simulink model "sm_cable_robot"  (R2021b)
settings: Solver=ode45  StartTime=0.0  StopTime=10  MaxStep=0.01  RelTol=1e-3  EnableMultiTasking=on
model workspace: external: MATLAB File sm_cable_robot_parameters.m (data not in the file)
values from neighbouring files (symbols this model uses):
  g = 9.80665    [sm_cable_robot_parameters.m]
undefined symbols (not defined in the file or in its folder): ball, frame, Hand, Left, mover, Right, X, Y, Z
libraries: sm_lib x12, nesl_utility x7, sm_cable_robot_lib x4
Description:
  | Cable Robot
settings Model: Creator=The MathWorks, Inc.  LastModifiedBy=The MathWorks, Inc.
settings SolverCC: AlgebraicLoopSolver=TrustRegion  MinimalZcImpactIntegration=on
settings DataIOCC: LimitDataPoints=on  ReturnWorkspaceOutputs=off
settings OptimizationCC: LifeSpan=inf
settings DebuggingCC: AllowSymbolicDim=off  SFUnexpectedBacktrackingDiag=warning  SFNoUnconditionalDefaultTransitionDiag=warning  SFExecutionAtInitializationDiag=none  SFMachineParentedDataDiag=warning  ArithmeticOperatorsInVariantConditions=warning
settings SFSimCC: SimUseLocalCustomCode=off
settings RTWCC: RTWUseLocalCustomCode=off
settings CodeAppCC: StateflowObjectComments=on
settings GRTTargetCC: TargetLangStandard=C89/C90 (ANSI)
settings ConfigComp: CovMetricSettings=dw  CovSaveCumulativeToWorkspaceVar=on  CovSaveSingleToWorkspaceVar=on  CovExternalEMLEnable=off  CovSFcnEnable=off
settings SimscapeCC: SimscapeNominalValues="[{\"value\":\"10\",\"unit\":\"V\"},{\"value\":\"1\",\"unit\":\"A\"},{\"value\":\"10\",\"unit\":\"N*m\"},{\"value\":\"10\",\"unit\":\"bar\"},{\"value\":\"100\",\"unit\":\"kJ/kg\"},{\"value\":\"1\",\"unit\":\"kW\"},{\"value\":\"300\",\"unit\":\"K\"},{\"value\":\"100\",\"unit\":\"cm^3/s\"},{\"value\":\"1\",\"unit\":\"kN\"},{\"value\":\"1\",\"unit\":\"g/cm^3\"},{\"value\":\"1\",\"unit\":\"l\"},{\"value\":\"1\",\"unit\":\"cm^2\"},{\"value\":\"60\",\"unit\":\"Hz\"}]"  SimscapeLogType=all  SimscapeLogName=simlog_sm_cable_robot  SimscapeLogDataHistory=10000
settings ConfigurationSet: Description=SimMechanics 2G
settings DiagnosticsConfigSet: SimMechanicsRigidlyBoundBlock=none
settings ExplorerConfigSet: InternalSimMechanicsExplorerSettings="<ExplorerConfiguration><canonicalview>default</canonicalview><AnimationSetting><BasePlaybackSpeed>1.0</BasePlaybackSpeed><PlaybackSpeedFactor>0.5</PlaybackSpeedFactor></AnimationSetting><TilePanel><TileInfo><Tiles Columns=\"2\" Count=\"4\" Rows=\"2\"><Column Weight=\"0.4996\"/><Column Weight=\"0.5004\"/><Row Weight=\"0.5\"/><Row Weight=\"0.5\"/><Tile Height=\"1\" Width=\"1\" X=\"0\" Y=\"0\"/><Tile Height=\"1\" Width=\"1\" X=\"0\" Y=\"1\"/><Tile Height=\"1\" Width=\"1\" X=\"1\" Y=\"0\"/><Tile Height=\"1\" Width=\"1\" X=\"1\" Y=\"1\"/></Tiles></TileInfo><SceneInfo><SceneViewer><BGColor><R>0.60000002384185791</R><G>0.60000002384185791</G><B>0.60000002384185791</B></BGColor><Camera><DoPerspective>on</DoPerspective><Position><X>0</X><Y>0</Y><Z>1.80000000000000004</Z></Position><Center><X>0</X><Y>0</Y><Z>0.6835266900559267</Z></Center><Up><X>0</X><Y>1</Y><Z>0</Z></Up><ViewLimDist>1</ViewLimDist><YLim>0.466307658154998583</YLim><XLim>0.599116801300409563</XLim></Camera></SceneViewer><SceneViewer><BGColor><R>0.60000002384185791</R><G>0.60000002384185791</G><B>0.60000002384185791</B></BGColor><Camera><DoPerspective>on</DoPerspective><Position><X>-0.869999999999999996</X><Y>-0.719999999999999973</Y><Z>1</Z></Position><Center><X>0.720937841330330564</X><Y>0.696383532720419751</Y><Z>0.00254680794336636929</Z></Center><Up><X>0.316740818644561883</X><Y>0.281988691207070763</Y><Z>0.905625547252116636</Z></Up><ViewLimDist>1</ViewLimDist><YLim>0.466307658154998583</YLim><XLim>0.599116801300409563</XLim></Camera></SceneViewer><SceneViewer><BGColor><R>0.60000002384185791</R><G>0.60000002384185791</G><B>0.60000002384185791</B></BGColor><Camera><DoPerspective>on</DoPerspective><Position><X>2.03939800918097314</X><Y>9.95798776770584482e-09</Y><Z>0.494999989241745375</Z></Position><Center><X>0.644699031710575188</X><Y>9.95798776770584482e-09</Y><Z>0.494999989241745375</Z></Center><Up><X>-0</X><Y>0</Y><Z>1</Z></Up><ViewLimDist>1</ViewLimDist><YLim>0.466307658154998583</YLim><XLim>0.599116801300409563</XLim></Camera></SceneViewer><SceneViewer><BGColor><R>0.60000002384185791</R><G>0.60000002384185791</G><B>0.60000002384185791</B></BGColor><Camera><DoPerspective>on</DoPerspective><Position><X>1.69344100606403369</X><Y>-0.966528451082007023</Y><Z>0.938335299313491245</Z></Position><Center><X>0.749070842638739132</X><Y>-0.395339740352455893</Y><Z>0.516094349779432804</Z></Center><Up><X>-0.304859850331606563</X><Y>0.186390498904929286</Y><Z>0.933980221189807835</Z></Up><ViewLimDist>1</ViewLimDist><YLim>0.466307658154998583</YLim><XLim>0.599116801300409563</XLim></Camera></SceneViewer></SceneInfo></TilePanel><MechEditorPanel><Cameras><Camera><Id>Camera1</Id><Value><Name>Overhead</Name><NativeCamera><PositionKeyframeSet><Keyframe><Time>+0.0000000000000000e+00</Time><Value><X>+0.0000000000000000e+00</X><Y>+0.0000000000000000e+00</Y><Z>+1.8000000000000000e+00</Z></Value></Keyframe></PositionKeyframeSet><CenterKeyframeSet><Keyframe><Time>+0.0000000000000000e+00</Time><Value><X>+0.0000000000000000e+00</X><Y>+0.0000000000000000e+00</Y><Z>+6.8352669005592670e-01</Z></Value></Keyframe></CenterKeyframeSet><UpVectorKeyframeSet><Keyframe><Time>+0.0000000000000000e+00</Time><Value><X>+0.0000000000000000e+00</X><Y>+1.0000000000000000e+00</Y><Z>+0.0000000000000000e+00</Z></Value></Keyframe></UpVectorKeyframeSet></NativeCamera></Value></Camera><Camera><Id>Camera2</Id><Value><Name>Swivel Pulley</Name><NativeCamera><PositionKeyframeSet><Keyframe><Time>+0.0000000000000000e+00</Time><Value><X>-8.7000000000000000e-01</X><Y>-7.1999999999999997e-01</Y><Z>+1.0000000000000000e+00</Z></Value></Keyframe></PositionKeyframeSet><CenterKeyframeSet><Keyframe><Time>+0.0000000000000000e+00</Time><Value><X>+7.2093784133033056e-01</X><Y>+6.9638353272041975e-01</Y><Z>+2.5468079433663693e-03</Z></Value></Keyframe></CenterKeyframeSet><UpVectorKeyframeSet><Keyframe><Time>+0.0000000000000000e+00</Time><Value><X>+3.1674081864456188e-01</X><Y>+2.8198869120707076e-01</Y><Z>+9.0562554725211664e-01</Z></Value></Keyframe></UpVectorKeyframeSet></NativeCamera></Value></Camera><Camera><Id>Camera3</Id><Value><Name>Flyover</Name><NativeCamera><PositionKeyframeSet><Keyframe><Time>+0.0000000000000000e+00</Time><Value><X>+1.6934410060640337e+00</X><Y>-9.6652845108200702e-01</Y><Z>+9.3833529931349124e-01</Z></Value></Keyframe><Keyframe><Time>+4.9990750394185373e+00</Time><Value><X>+8.7196584858736648e-01</X><Y>+7.5039304919046734e-01</Y><Z>+1.0201392219856453e+00</Z></Value></Keyframe><Keyframe><Time>+6.7557213998445649e+00</Time><Value><X>+1.0978317870949922e-01</X><Y>+1.0441353295504237e+00</Y><Z>+6.6281255365999214e-01</Z></Value></Keyframe><Keyframe><Time>+1.0000000000000000e+01</Time><Value><X>-1.7603692267125191e+00</X><Y>+1.0439399563553646e+00</Y><Z>+9.9074072437996419e-01</Z></Value></Keyframe></PositionKeyframeSet><CenterKeyframeSet><Keyframe><Time>+0.0000000000000000e+00</Time><Value><X>+7.4907084263873913e-01</X><Y>-3.9533974035245589e-01</Y><Z>+5.1609434977943280e-01</Z></Value></Keyframe><Keyframe><Time>+4.9990750394185373e+00</Time><Value><X>-3.2753521429289556e-02</X><Y>+1.9773238156433104e-01</Y><Z>+4.6145766220277656e-01</Z></Value></Keyframe><Keyframe><Time>+6.7557213998445649e+00</Time><Value><X>-1.3285810096836129e-01</X><Y>+7.6142497332660819e-02</Y><Z>+4.2339186817260011e-01</Z></Value></Keyframe><Keyframe><Time>+1.0000000000000000e+01</Time><Value><X>-7.4995691707333356e-01</X><Y>+3.6716342260572554e-01</Y><Z>+4.9700352462356229e-01</Z></Value></Keyframe></CenterKeyframeSet><UpVectorKeyframeSet><Keyframe><Time>+0.0000000000000000e+00</Time><Value><X>-3.0485985033160656e-01</X><Y>+1.8639049890492929e-01</Y><Z>+9.3398022118980784e-01</Z></Value></Keyframe><Keyframe><Time>+4.9990750394185373e+00</Time><Value><X>-3.9777312998695924e-01</X><Y>-2.4315087035137614e-01</Y><Z>+8.8467745043475932e-01</Z></Value></Keyframe><Keyframe><Time>+6.7557213998445649e+00</Time><Value><X>-1.1640564560715221e-01</X><Y>-2.1087616588642455e-01</Y><Z>+9.7055704022577838e-01</Z></Value></Keyframe><Keyframe><Time>+1.0000000000000000e+01</Time><Value><X>+3.1157098740679545e-01</X><Y>-2.1078784768502751e-01</Y><Z>+9.2654843536356379e-01</Z></Value></Keyframe></UpVectorKeyframeSet></NativeCamera></Value></Camera><Camera><Id>Camera4</Id><Value><Name>Side</Name><NativeCamera><PositionKeyframeSet><Keyframe><Time>+0.0000000000000000e+00</Time><Value><X>+2.0393980091809731e+00</X><Y>+9.9579877677058448e-09</Y><Z>+4.9499998924174538e-01</Z></Value></Keyframe></PositionKeyframeSet><CenterKeyframeSet><Keyframe><Time>+0.0000000000000000e+00</Time><Value><X>+6.4469903171057519e-01</X><Y>+9.9579877677058448e-09</Y><Z>+4.9499998924174538e-01</Z></Value></Keyframe></CenterKeyframeSet><UpVectorKeyframeSet><Keyframe><Time>+0.0000000000000000e+00</Time><Value><X>-0.0000000000000000e+00</X><Y>+0.0000000000000000e+00</Y><Z>+1.0000000000000000e+00</Z></Value></Keyframe></UpVectorKeyframeSet></NativeCamera></Value></Camera></Cameras><GfxPanelCameraMap><MapElement CameraMLId=\"Camera1\" GfxPanelIndex=\"0\"/><MapElement CameraMLId=\"Camera2\" GfxPanelIndex=\"1\"/><MapElement CameraMLId=\"Camera4\" GfxPanelIndex=\"2\"/><MapElement CameraMLId=\"Camera3\" GfxPanelIndex=\"3\"/></GfxPanelCameraMap><VideoCreator><PlaybackSpeedRatio>1.0</PlaybackSpeedRatio><FrameRate>30</FrameRate><VideoFormat>Motion JPEG AVI</VideoFormat><FrameSize>auto</FrameSize></VideoCreator></MechEditorPanel></ExplorerConfiguration>"

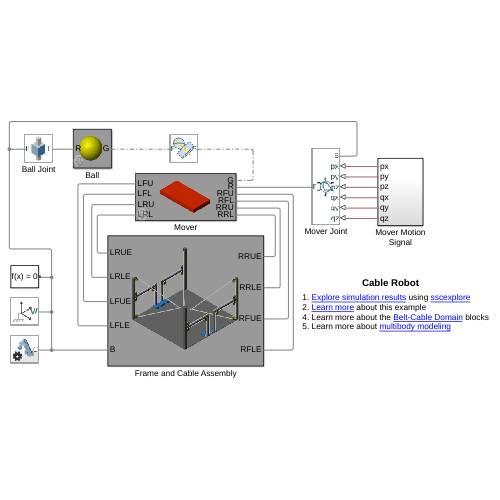
[thumbnail: Simulink's stored preview of the top-level diagram]
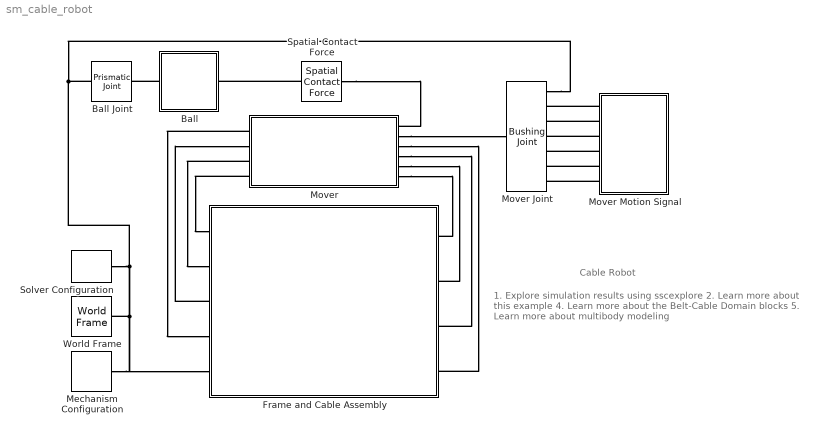
== system sm_cable_robot ==
  note: 1. Explore simulation results using sscexplore
      | 2. Learn more about this example
      | 4. Learn more about the Belt-Cable Domain blocks
      | 5. Learn more about multibody modeling
  note: Cable Robot
  Ball : Subsystem  mask(Ball){radius=ball.radius, mass=ball.mass, color=ball.color}
      mask prompts: mass "Mass (kg)"; color "Color [r g b]"
      mask help:
      | This block models the ball of the cable robot. It is modeled as a thin walled hollow sphere.
      |
      | Port R corresponds to the origin of the ball.
      mask init:
      | inertia = (2/3) * mass * radius ^ 2;
      | 
      | moments = [inertia inertia inertia];
      mask DialogControl Tab1 Prompt: Dimensions
      mask DialogControl Tab2 Prompt: Material Properties
      mask Display: image(fullfile(matlabroot,'toolbox','physmod','sm','smdemos','cable_robot','images','sm_cable_robot_ball.png'));
  Ball Joint : sm_lib/Joints/Prismatic Joint  JointMode=Normal  SenseConstraintForce=off  SenseConstraintForceX=off  SenseConstraintForceY=off  SenseConstraintForceZ=off  SenseConstraintTorque=off  SenseConstraintTorqueX=off  SenseConstraintTorqueY=off  SenseConstraintTorqueZ=off  SenseTotalForce=off  SenseTotalForceX=off  SenseTotalForceY=off  SenseTotalForceZ=off  SenseTotalTorque=off  SenseTotalTorqueX=off  SenseTotalTorqueY=off  SenseTotalTorqueZ=off  CompositeWrenchDir=FollowerOnBase  CompositeWrenchFrame=BaseFrame  EquilibriumPosition=0  EquilibriumPositionUnits=m  SpringStiffness=0  SpringStiffnessUnits=N/m  DampingCoefficient=0  DampingCoefficientUnits=N/(m/s)  TorqueActuationMode=NoTorque  MotionActuationMode=ComputedMotion  SensePosition=off  SenseVelocity=off  SenseAcceleration=off  SenseTorqueForce=off  SenseLowerLimitTorqueForce=off  SenseUpperLimitTorqueForce=off  LowerLimitSpecify=off  LowerLimitBound=-1  LowerLimitBoundUnits=m  LowerLimitStiffness=1e6  LowerLimitStiffnessUnits=N/m  LowerLimitDamping=1e3  LowerLimitDampingUnits=N/(m/s)  LowerLimitTransitionRegionWidth=1e-4  LowerLimitTransitionRegionWidthUnits=m  UpperLimitSpecify=off  UpperLimitBound=1  UpperLimitBoundUnits=m  UpperLimitStiffness=1e6  UpperLimitStiffnessUnits=N/m  UpperLimitDamping=1e3  UpperLimitDampingUnits=N/(m/s)  UpperLimitTransitionRegionWidth=1e-4  UpperLimitTransitionRegionWidthUnits=m  PositionTargetSpecify=on  PositionTargetPriority=High  PositionTargetValue=ball.pz0  PositionTargetValueUnits=m  VelocityTargetSpecify=off  VelocityTargetPriority=High  VelocityTargetValue=0  VelocityTargetValueUnits=m/s
  Frame and Cable Assembly : Subsystem
      mask Display: image(fullfile(matlabroot,'toolbox','physmod','sm','smdemos','cable_robot','images','sm_cable_robot_frame_cable_assembly_whole.png'));
  Mechanism Configuration : sm_lib/Utilities/Mechanism Configuration  UniformGravity=Constant  GravityVector=[0 0 -g]  GravityUnits=m/s^2  LinearizationDelta=0.001  JointModeTransitionNonlinearIterations=2
  Mover : Subsystem  mask(Mover){width=mover.width, length=mover.length, thickness=mover.thickness, connectorOffset=mover.connectorOffset, rho=mover.density, color=mover.color}
      mask prompts: width "Width (m)"; length "Length (m)"; thickness "Thickness (m)"; connectorOffset "Connector Offset (m)"; rho "Density (kg/m^3)"; color "Color [r g b]"
      mask help:
      | This block models the mover of the cable robot. It is a simple plate with attachment points at the corners for the cables.
      |
      | Port R corresponds to the center point of the mover solid. The remaining points correspond to the attachment points for the cables.
      mask init:
      | dimension = [width length thickness];
      mask DialogControl Tab1 Prompt: Dimensions
      mask DialogControl Tab2 Prompt: Material Properties
      mask Display: image(fullfile(matlabroot,'toolbox','physmod','sm','smdemos','cable_robot','images','sm_cable_robot_mover.png'));
  Mover Joint : sm_lib/Joints/Bushing Joint  JointMode=Normal  SenseConstraintForce=off  SenseConstraintForceX=off  SenseConstraintForceY=off  SenseConstraintForceZ=off  SenseConstraintTorque=off  SenseConstraintTorqueX=off  SenseConstraintTorqueY=off  SenseConstraintTorqueZ=off  SenseTotalForce=off  SenseTotalForceX=off  SenseTotalForceY=off  SenseTotalForceZ=off  SenseTotalTorque=off  SenseTotalTorqueX=off  SenseTotalTorqueY=off  SenseTotalTorqueZ=off  CompositeWrenchDir=FollowerOnBase  CompositeWrenchFrame=BaseFrame  PxEquilibriumPosition=0  PxEquilibriumPositionUnits=m  PxSpringStiffness=0  PxSpringStiffnessUnits=N/m  PxDampingCoefficient=0  PxDampingCoefficientUnits=N/(m/s)  PxTorqueActuationMode=ComputedTorque  PxMotionActuationMode=InputMotion  PxSensePosition=off  PxSenseVelocity=off  PxSenseAcceleration=off  PxSenseTorqueForce=off  PxSenseLowerLimitTorqueForce=off  PxSenseUpperLimitTorqueForce=off  PxLowerLimitSpecify=off  PxLowerLimitBound=-1  PxLowerLimitBoundUnits=m  PxLowerLimitStiffness=1e6  PxLowerLimitStiffnessUnits=N/m  PxLowerLimitDamping=1e3  PxLowerLimitDampingUnits=N/(m/s)  PxLowerLimitTransitionRegionWidth=1e-4  PxLowerLimitTransitionRegionWidthUnits=m  PxUpperLimitSpecify=off  PxUpperLimitBound=1  PxUpperLimitBoundUnits=m  PxUpperLimitStiffness=1e6  PxUpperLimitStiffnessUnits=N/m  PxUpperLimitDamping=1e3  PxUpperLimitDampingUnits=N/(m/s)  PxUpperLimitTransitionRegionWidth=1e-4  PxUpperLimitTransitionRegionWidthUnits=m  PxPositionTargetSpecify=on  PxPositionTargetPriority=High  PxPositionTargetValue=mover.motionSignal.px0  PxPositionTargetValueUnits=m  PxVelocityTargetSpecify=off  PxVelocityTargetPriority=High  PxVelocityTargetValue=0  PxVelocityTargetValueUnits=m/s  PyEquilibriumPosition=0  PyEquilibriumPositionUnits=m  PySpringStiffness=0  PySpringStiffnessUnits=N/m  PyDampingCoefficient=0  PyDampingCoefficientUnits=N/(m/s)  PyTorqueActuationMode=ComputedTorque  PyMotionActuationMode=InputMotion  PySensePosition=off  PySenseVelocity=off  PySenseAcceleration=off  PySenseTorqueForce=off  PySenseLowerLimitTorqueForce=off  PySenseUpperLimitTorqueForce=off  PyLowerLimitSpecify=off  PyLowerLimitBound=-1  PyLowerLimitBoundUnits=m  PyLowerLimitStiffness=1e6  PyLowerLimitStiffnessUnits=N/m  PyLowerLimitDamping=1e3  PyLowerLimitDampingUnits=N/(m/s)  PyLowerLimitTransitionRegionWidth=1e-4  PyLowerLimitTransitionRegionWidthUnits=m  PyUpperLimitSpecify=off  PyUpperLimitBound=1  PyUpperLimitBoundUnits=m  PyUpperLimitStiffness=1e6  PyUpperLimitStiffnessUnits=N/m  PyUpperLimitDamping=1e3  PyUpperLimitDampingUnits=N/(m/s)  PyUpperLimitTransitionRegionWidth=1e-4  PyUpperLimitTransitionRegionWidthUnits=m  PyPositionTargetSpecify=on  PyPositionTargetPriority=High  PyPositionTargetValue=mover.motionSignal.py0  PyPositionTargetValueUnits=m  PyVelocityTargetSpecify=off  PyVelocityTargetPriority=High  PyVelocityTargetValue=0  PyVelocityTargetValueUnits=m/s  PzEquilibriumPosition=0  PzEquilibriumPositionUnits=m  PzSpringStiffness=0  PzSpringStiffnessUnits=N/m  PzDampingCoefficient=0  PzDampingCoefficientUnits=N/(m/s)  PzTorqueActuationMode=ComputedTorque  PzMotionActuationMode=InputMotion  PzSensePosition=off  PzSenseVelocity=off  PzSenseAcceleration=off  PzSenseTorqueForce=off  PzSenseLowerLimitTorqueForce=off  PzSenseUpperLimitTorqueForce=off  PzLowerLimitSpecify=off  PzLowerLimitBound=-1  PzLowerLimitBoundUnits=m  PzLowerLimitStiffness=1e6  PzLowerLimitStiffnessUnits=N/m  PzLowerLimitDamping=1e3  PzLowerLimitDampingUnits=N/(m/s)  PzLowerLimitTransitionRegionWidth=1e-4  PzLowerLimitTransitionRegionWidthUnits=m  PzUpperLimitSpecify=off  PzUpperLimitBound=1  PzUpperLimitBoundUnits=m  PzUpperLimitStiffness=1e6  PzUpperLimitStiffnessUnits=N/m  PzUpperLimitDamping=1e3  PzUpperLimitDampingUnits=N/(m/s)  PzUpperLimitTransitionRegionWidth=1e-4  PzUpperLimitTransitionRegionWidthUnits=m  PzPositionTargetSpecify=on  PzPositionTargetPriority=High  PzPositionTargetValue=mover.motionSignal.pz0  PzPositionTargetValueUnits=m  PzVelocityTargetSpecify=off  PzVelocityTargetPriority=High  PzVelocityTargetValue=0  PzVelocityTargetValueUnits=m/s  RxEquilibriumPosition=0  RxEquilibriumPositionUnits=deg  RxSpringStiffness=0  RxSpringStiffnessUnits=N*m/deg  RxDampingCoefficient=0  RxDampingCoefficientUnits=N*m/(deg/s)  RxTorqueActuationMode=ComputedTorque  RxMotionActuationMode=InputMotion  RxSensePosition=off  RxSenseVelocity=off  RxSenseAcceleration=off  RxSenseTorqueForce=off  RxSenseLowerLimitTorqueForce=off  RxSenseUpperLimitTorqueForce=off  RxLowerLimitSpecify=off  RxLowerLimitBound=-90  RxLowerLimitBoundUnits=deg  RxLowerLimitStiffness=1e4  RxLowerLimitStiffnessUnits=N*m/deg  RxLowerLimitDamping=10  RxLowerLimitDampingUnits=N*m/(deg/s)  RxLowerLimitTransitionRegionWidth=0.1  RxLowerLimitTransitionRegionWidthUnits=deg  RxUpperLimitSpecify=off  RxUpperLimitBound=90  RxUpperLimitBoundUnits=deg  RxUpperLimitStiffness=1e4  RxUpperLimitStiffnessUnits=N*m/deg  RxUpperLimitDamping=10  RxUpperLimitDampingUnits=N*m/(deg/s)  RxUpperLimitTransitionRegionWidth=0.1  RxUpperLimitTransitionRegionWidthUnits=deg  RxPositionTargetSpecify=on  RxPositionTargetPriority=High  RxPositionTargetValue=0  RxPositionTargetValueUnits=deg  RxVelocityTargetSpecify=off  RxVelocityTargetPriority=High  RxVelocityTargetValue=0  RxVelocityTargetValueUnits=deg/s  RyEquilibriumPosition=0  RyEquilibriumPositionUnits=deg  RySpringStiffness=0  RySpringStiffnessUnits=N*m/deg  RyDampingCoefficient=0  RyDampingCoefficientUnits=N*m/(deg/s)  RyTorqueActuationMode=ComputedTorque  RyMotionActuationMode=InputMotion  RySensePosition=off  RySenseVelocity=off  RySenseAcceleration=off  RySenseTorqueForce=off  RySenseLowerLimitTorqueForce=off  RySenseUpperLimitTorqueForce=off  RyLowerLimitSpecify=off  RyLowerLimitBound=-90  RyLowerLimitBoundUnits=deg  RyLowerLimitStiffness=1e4  RyLowerLimitStiffnessUnits=N*m/deg  RyLowerLimitDamping=10  RyLowerLimitDampingUnits=N*m/(deg/s)  RyLowerLimitTransitionRegionWidth=0.1  RyLowerLimitTransitionRegionWidthUnits=deg  RyUpperLimitSpecify=off  RyUpperLimitBound=90  RyUpperLimitBoundUnits=deg  RyUpperLimitStiffness=1e4  RyUpperLimitStiffnessUnits=N*m/deg  RyUpperLimitDamping=10  RyUpperLimitDampingUnits=N*m/(deg/s)  RyUpperLimitTransitionRegionWidth=0.1  RyUpperLimitTransitionRegionWidthUnits=deg  RyPositionTargetSpecify=on  RyPositionTargetPriority=High  RyPositionTargetValue=0  RyPositionTargetValueUnits=deg  RyVelocityTargetSpecify=off  RyVelocityTargetPriority=High  RyVelocityTargetValue=0  RyVelocityTargetValueUnits=deg/s  RzEquilibriumPosition=0  RzEquilibriumPositionUnits=deg  RzSpringStiffness=0  RzSpringStiffnessUnits=N*m/deg  RzDampingCoefficient=0  RzDampingCoefficientUnits=N*m/(deg/s)  RzTorqueActuationMode=ComputedTorque  RzMotionActuationMode=InputMotion  RzSensePosition=off  RzSenseVelocity=off  RzSenseAcceleration=off  RzSenseTorqueForce=off  RzSenseLowerLimitTorqueForce=off  RzSenseUpperLimitTorqueForce=off  RzLowerLimitSpecify=off  RzLowerLimitBound=-90  RzLowerLimitBoundUnits=deg  RzLowerLimitStiffness=1e4  RzLowerLimitStiffnessUnits=N*m/deg  RzLowerLimitDamping=10  RzLowerLimitDampingUnits=N*m/(deg/s)  RzLowerLimitTransitionRegionWidth=0.1  RzLowerLimitTransitionRegionWidthUnits=deg  RzUpperLimitSpecify=off  RzUpperLimitBound=90  RzUpperLimitBoundUnits=deg  RzUpperLimitStiffness=1e4  RzUpperLimitStiffnessUnits=N*m/deg  RzUpperLimitDamping=10  RzUpperLimitDampingUnits=N*m/(deg/s)  RzUpperLimitTransitionRegionWidth=0.1  RzUpperLimitTransitionRegionWidthUnits=deg  RzPositionTargetSpecify=on  RzPositionTargetPriority=High  RzPositionTargetValue=0  RzPositionTargetValueUnits=deg  RzVelocityTargetSpecify=off  RzVelocityTargetPriority=High  RzVelocityTargetValue=0  RzVelocityTargetValueUnits=deg/s
  Mover Motion Signal : Subsystem
  Solver Configuration : nesl_utility/Solver Configuration  PhysicalDomain=network_engine_domain  SubClassName=solver  LeftPortType=input  RightPortType=generic  Tones=[]  Harmonics=[]  SimulateNoise=off  Profile=off  UseLocalSampling=off  EnableSwitchedLinearOptims=on  FrequencyDomain=off  UseCCode=off  RelTol=0.001  AbsTol=1e-06  MinStep=1e-09  ToWorkspace=off  RevertToSquareIcSolve=off  NumHomotopyIterations=100  PhasorMode=off  PhasorModeNumHarmonics=1  DoDC=off  ResidualTolerance=1e-09  UseLocalSolver=off  LocalSolverChoice=NE_BACKWARD_EULER_ADVANCER  LocalSolverSampleTime=0.001  DoFixedCost=off  MaxNonlinIter=3  MaxModeIter=2  ComputeImpulses=off  ImpulseIterations=2  LinearAlgebra=Sparse  EquationFormulation=NE_TIME_EF  DelaysMemoryBudget=1024  AutomaticFiltering=on  FilteringTimeConstant=0.001  PartitionStorageMethod=AS_NEEDED  PartitionMemoryBudget=1024  PartitionMethod=FAST
      settings: SourceProductBaseCode=PW,SS
  Spatial Contact Force : sm_lib/Forces and Torques/Spatial Contact Force  CoefficientOfDynamicFriction=0.1  CoefficientOfStaticFriction=0.25  SenseContactBaseRotation=off  SenseContactBaseTranslation=off  NormalDamping=0  NormalDampingUnits=N/(m/s)  SenseContactFollowerRotation=off  SenseContactFollowerTranslation=off  SenseContactSignal=off  NormalStiffness=contact.stiffness  NormalStiffnessUnits=N/m  FrictionalCriticalVelocity=1e-2  FrictionalCriticalVelocityUnits=m/s  ZeroCrossDetectContactStartAndEnd=on  FrictionType=None  SenseFrictionalForceMagnitude=off  SenseNormalForceMagnitude=off  NormalForceType=SmoothSpringDamper  SenseNormalVelocity=off  SenseSeparationDistance=off  SenseTangentialVelocity=off  SenseTangentialVelocityMagnitude=off  NormalTransitionRegionWidth=contact.transRegWidth  NormalTransitionRegionWidthUnits=m
  World Frame : sm_lib/Frames and Transforms/World Frame
  connections:
  Solver Configuration/RConn1 -- Frame and Cable Assembly/LConn5 -- Mechanism Configuration/RConn1 -- World Frame/RConn1 -- Mover Joint/LConn1 -- Ball Joint/LConn1
  Mover/RConn2 -- Mover Joint/RConn1
  Ball/LConn1 -- Ball Joint/RConn1
  Mover Motion Signal/RConn1 -- Mover Joint/LConn2
  Mover Motion Signal/RConn2 -- Mover Joint/LConn3
  Mover Motion Signal/RConn3 -- Mover Joint/LConn4
  Mover Motion Signal/RConn4 -- Mover Joint/LConn5
  Mover Motion Signal/RConn5 -- Mover Joint/LConn6
  Mover Motion Signal/RConn6 -- Mover Joint/LConn7
  Mover/LConn1 -- Frame and Cable Assembly/LConn4
  Mover/RConn3 -- Frame and Cable Assembly/RConn4
  Frame and Cable Assembly/LConn3 -- Mover/LConn2
  Mover/RConn4 -- Frame and Cable Assembly/RConn3
  Mover/LConn3 -- Frame and Cable Assembly/LConn2
  Mover/RConn5 -- Frame and Cable Assembly/RConn2
  Mover/LConn4 -- Frame and Cable Assembly/LConn1
  Mover/RConn6 -- Frame and Cable Assembly/RConn1
  Spatial Contact Force/RConn1 -- Ball/RConn1
  Spatial Contact Force/LConn1 -- Mover/RConn1

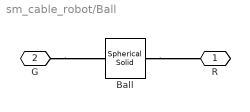
== system sm_cable_robot/Ball ==
  Ball : sm_lib/Body Elements/Spherical Solid  GraphicAmbientColor=[0.15 0.15 0.15 1.0]  BasedOnType=Density  CenterOfMass=[0 0 0]  CenterOfMassUnits=m  GraphicDiffuseColor=color  Density=1000  DensityUnits=kg/m^3  DoExposeReferenceFrame=on  GraphicEmissiveColor=[0.0 0.0 0.0 1.0]  ExportEntireGeometry=on  SerializedExposedGeometries=<ExposedGeometries><ExposedGeometry><RawGeometryId>entire</RawGeometryId><ExposedGeometryId>G</ExposedGeometryId></ExposedGeometry></ExposedGeometries>  SerializedFrames=<Frames/>  MarkerShape=Sphere  MarkerSize=10  GraphicType=FromGeometry  InertiaType=Custom  Mass=mass  MassUnits=kg  MomentsOfInertia=moments  MomentsOfInertiaUnits=kg*m^2  GraphicOpacity=1.0  ProductsOfInertia=[0 0 0]  ProductsOfInertiaUnits=kg*m^2  GraphicShininess=75  GraphicSpecularColor=[0.5 0.5 0.5 1.0]  SphereRadius=radius  SphereRadiusUnits=m  GraphicVisPropType=SimpleVisualProperties
  R : PMIOPort  Side=Left
  G : PMIOPort  Port=2  Side=Right
  connections:
  Ball/RConn1 -- R/RConn1
  G/RConn1 -- Ball/LConn1

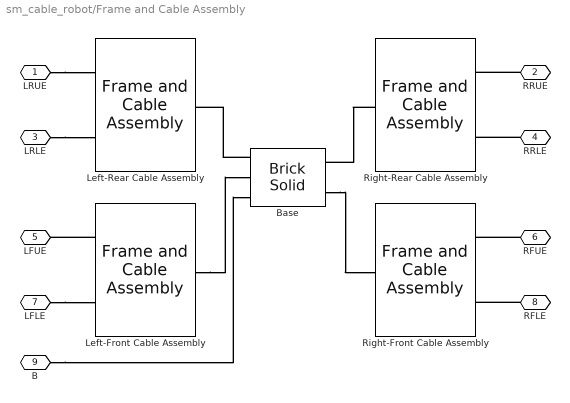
== system sm_cable_robot/Frame and Cable Assembly ==
  Base : sm_lib/Body Elements/Brick Solid  GraphicAmbientColor=[0.15 0.15 0.15 1.0]  BasedOnType=Density  BrickDimensions=[frame.baseWidth frame.baseWidth frame.baseThickness]  BrickDimensionUnits=m  CenterOfMass=[0 0 0]  CenterOfMassUnits=m  GraphicDiffuseColor=frame.color  Density=frame.density  DensityUnits=kg/m^3  DoExposeReferenceFrame=off  GraphicEmissiveColor=[0.0 0.0 0.0 1.0]  ExportEntireGeometry=off  SerializedFrames=<Frames><Frame><Id>Frame3</Id><Value><Name>LR</Name><Origin><Source>GeometricFeature</Source><FeatureName>-x +y +z point</FeatureName></Origin><PrimaryAxis><DefinedDirection>+Y</DefinedDirection><Source>ReferenceFrame</Source><SourceDirection>-Y</SourceDirection><FeatureName></FeatureName></PrimaryAxis><SecondaryAxis><DefinedDirection>+Z</DefinedDirection><Source>ReferenceFrame</Source><SourceDirection>+Z</SourceDirection><FeatureName></FeatureName></SecondaryAxis></Value></Frame><Frame><Id>Frame4</Id><Value><Name>RR</Name><Origin><Source>GeometricFeature</Source><FeatureName>+x +y +z point</FeatureName></Origin><PrimaryAxis><DefinedDirection>+Z</DefinedDirection><Source>ReferenceFrame</Source><SourceDirection>+Z</SourceDirection><FeatureName></FeatureName></PrimaryAxis><SecondaryAxis><DefinedDirection>+X</DefinedDirection><Source>ReferenceFrame</Source><SourceDirection>-X</SourceDirection><FeatureName></FeatureName></SecondaryAxis></Value></Frame><Frame><Id>Frame5</Id><Value><Name>LF</Name><Origin><Source>GeometricFeature</Source><FeatureName>-x -y +z point</FeatureName></Origin><PrimaryAxis><DefinedDirection>+Z</DefinedDirection><Source>ReferenceFrame</Source><SourceDirection>+Z</SourceDirection><FeatureName></FeatureName></PrimaryAxis><SecondaryAxis><DefinedDirection>+X</DefinedDirection><Source>ReferenceFrame</Source><SourceDirection>+X</SourceDirection><FeatureName></FeatureName></SecondaryAxis></Value></Frame><Frame><Id>Frame6</Id><Value><Name>RF</Name><Origin><Source>GeometricFeature</Source><FeatureName>+x -y +z point</FeatureName></Origin><PrimaryAxis><DefinedDirection>+Z</DefinedDirection><Source>ReferenceFrame</Source><SourceDirection>+Z</SourceDirection><FeatureName></FeatureName></PrimaryAxis><SecondaryAxis><DefinedDirection>+X</DefinedDirection><Source>ReferenceFrame</Source><SourceDirection>+X</SourceDirection><FeatureName></FeatureName></SecondaryAxis></Value></Frame><Frame><Id>Frame7</Id><Value><Name>B</Name><Origin><Source>GeometricFeature</Source><FeatureName>+z surface</FeatureName></Origin><PrimaryAxis><DefinedDirection>+Z</DefinedDirection><Source>ReferenceFrame</Source><SourceDirection>+Z</SourceDirection><FeatureName></FeatureName></PrimaryAxis><SecondaryAxis><DefinedDirection>+X</DefinedDirection><Source>ReferenceFrame</Source><SourceDirection>+X</SourceDirection><FeatureName></FeatureName></SecondaryAxis></Value></Frame></Frames>  MarkerShape=Sphere  MarkerSize=10  GraphicType=FromGeometry  InertiaType=CalculateFromGeometry  Mass=1  MassUnits=kg  MomentsOfInertia=[1 1 1]  MomentsOfInertiaUnits=kg*m^2  GraphicOpacity=1.0  ProductsOfInertia=[0 0 0]  ProductsOfInertiaUnits=kg*m^2  GraphicShininess=75  GraphicSpecularColor=[0.5 0.5 0.5 1.0]  GraphicVisPropType=SimpleVisualProperties
  Left-Front Cable Assembly : sm_cable_robot_lib/Frame and Cable Assembly  frameType=Left-Hand  frameColumnWidth=frame.columnWidth  frameColumnHeight=frame.columnHeight  frameBeamWidth=frame.beamWidth  frameBeamLength=frame.beamLength  bracketWidth=bracket.width  bracketThickness=bracket.thickness  bracketTolerance=bracket.tolerance  swivelHoleRadius=bracket.swivelHoleRadius  rightBracketWidth=bracket.rightBracketWidth  motorWidth=motor.width  motorHeight=motor.height  motorDepth=motor.depth  motorShaftRadius=motor.shaftRadius  motorShaftLength=motor.shaftLength  pulleyRadius=pulley.radius  pulleyThickness=pulley.thickness  pulleyHoleRadius=pulley.holeRadius  pulleyGrooveDepth=pulley.grooveDepth  pulleyGrooveWidth=pulley.grooveWidth  pulleyGrooveAngle=pulley.grooveAngle  pulleyFrameGap=pulley.frameGap  spoolRadius=spool.radius  spoolThickness=spool.thickness  spoolGrooveDepth=spool.grooveDepth  spoolGrooveWidth=spool.grooveWidth  spoolGrooveAngle=spool.grooveAngle  ringMajorRadius=ring.majorRadius  ringMinorRadius=ring.minorRadius  frameRho=frame.density  pinRho=frame.pinDensity  motorHousingRho=motor.housingDensity  motorShaftRho=motor.shaftDensity  pulleyRho=pulley.density  spoolRho=spool.density  ringRho=ring.density  frameColor=frame.color  bracketColor=bracket.color  pinColor=frame.pinColor  motorHousingColor=motor.housingColor  motorFlangeColor=motor.flangeColor  motorShaftColor=motor.shaftColor  pulleyColor=pulley.color  pulleyMarkerColor=pulley.markerColor  spoolColor=spool.color  spoolMarkerColor=spool.markerColor  cableColor=cable.color  ringColor=ring.color
      settings: SourceProductBaseCode=MS
  Left-Rear Cable Assembly : sm_cable_robot_lib/Frame and Cable Assembly  frameType=Right-Hand  frameColumnWidth=frame.columnWidth  frameColumnHeight=frame.columnHeight  frameBeamWidth=frame.beamWidth  frameBeamLength=frame.beamLength  bracketWidth=bracket.width  bracketThickness=bracket.thickness  bracketTolerance=bracket.tolerance  swivelHoleRadius=bracket.swivelHoleRadius  rightBracketWidth=bracket.rightBracketWidth  motorWidth=motor.width  motorHeight=motor.height  motorDepth=motor.depth  motorShaftRadius=motor.shaftRadius  motorShaftLength=motor.shaftLength  pulleyRadius=pulley.radius  pulleyThickness=pulley.thickness  pulleyHoleRadius=pulley.holeRadius  pulleyGrooveDepth=pulley.grooveDepth  pulleyGrooveWidth=pulley.grooveWidth  pulleyGrooveAngle=pulley.grooveAngle  pulleyFrameGap=pulley.frameGap  spoolRadius=spool.radius  spoolThickness=spool.thickness  spoolGrooveDepth=spool.grooveDepth  spoolGrooveWidth=spool.grooveWidth  spoolGrooveAngle=spool.grooveAngle  ringMajorRadius=ring.majorRadius  ringMinorRadius=ring.minorRadius  frameRho=frame.density  pinRho=frame.pinDensity  motorHousingRho=motor.housingDensity  motorShaftRho=motor.shaftDensity  pulleyRho=pulley.density  spoolRho=spool.density  ringRho=ring.density  frameColor=frame.color  bracketColor=bracket.color  pinColor=frame.pinColor  motorHousingColor=motor.housingColor  motorFlangeColor=motor.flangeColor  motorShaftColor=motor.shaftColor  pulleyColor=pulley.color  pulleyMarkerColor=pulley.markerColor  spoolColor=spool.color  spoolMarkerColor=spool.markerColor  cableColor=cable.color  ringColor=ring.color
      settings: SourceProductBaseCode=MS
  Right-Front Cable Assembly : sm_cable_robot_lib/Frame and Cable Assembly  frameType=Right-Hand  frameColumnWidth=frame.columnWidth  frameColumnHeight=frame.columnHeight  frameBeamWidth=frame.beamWidth  frameBeamLength=frame.beamLength  bracketWidth=bracket.width  bracketThickness=bracket.thickness  bracketTolerance=bracket.tolerance  swivelHoleRadius=bracket.swivelHoleRadius  rightBracketWidth=bracket.rightBracketWidth  motorWidth=motor.width  motorHeight=motor.height  motorDepth=motor.depth  motorShaftRadius=motor.shaftRadius  motorShaftLength=motor.shaftLength  pulleyRadius=pulley.radius  pulleyThickness=pulley.thickness  pulleyHoleRadius=pulley.holeRadius  pulleyGrooveDepth=pulley.grooveDepth  pulleyGrooveWidth=pulley.grooveWidth  pulleyGrooveAngle=pulley.grooveAngle  pulleyFrameGap=pulley.frameGap  spoolRadius=spool.radius  spoolThickness=spool.thickness  spoolGrooveDepth=spool.grooveDepth  spoolGrooveWidth=spool.grooveWidth  spoolGrooveAngle=spool.grooveAngle  ringMajorRadius=ring.majorRadius  ringMinorRadius=ring.minorRadius  frameRho=frame.density  pinRho=frame.pinDensity  motorHousingRho=motor.housingDensity  motorShaftRho=motor.shaftDensity  pulleyRho=pulley.density  spoolRho=spool.density  ringRho=ring.density  frameColor=frame.color  bracketColor=bracket.color  pinColor=frame.pinColor  motorHousingColor=motor.housingColor  motorFlangeColor=motor.flangeColor  motorShaftColor=motor.shaftColor  pulleyColor=pulley.color  pulleyMarkerColor=pulley.markerColor  spoolColor=spool.color  spoolMarkerColor=spool.markerColor  cableColor=cable.color  ringColor=ring.color
      settings: SourceProductBaseCode=MS
  Right-Rear Cable Assembly : sm_cable_robot_lib/Frame and Cable Assembly  frameType=Left-Hand  frameColumnWidth=frame.columnWidth  frameColumnHeight=frame.columnHeight  frameBeamWidth=frame.beamWidth  frameBeamLength=frame.beamLength  bracketWidth=bracket.width  bracketThickness=bracket.thickness  bracketTolerance=bracket.tolerance  swivelHoleRadius=bracket.swivelHoleRadius  rightBracketWidth=bracket.rightBracketWidth  motorWidth=motor.width  motorHeight=motor.height  motorDepth=motor.depth  motorShaftRadius=motor.shaftRadius  motorShaftLength=motor.shaftLength  pulleyRadius=pulley.radius  pulleyThickness=pulley.thickness  pulleyHoleRadius=pulley.holeRadius  pulleyGrooveDepth=pulley.grooveDepth  pulleyGrooveWidth=pulley.grooveWidth  pulleyGrooveAngle=pulley.grooveAngle  pulleyFrameGap=pulley.frameGap  spoolRadius=spool.radius  spoolThickness=spool.thickness  spoolGrooveDepth=spool.grooveDepth  spoolGrooveWidth=spool.grooveWidth  spoolGrooveAngle=spool.grooveAngle  ringMajorRadius=ring.majorRadius  ringMinorRadius=ring.minorRadius  frameRho=frame.density  pinRho=frame.pinDensity  motorHousingRho=motor.housingDensity  motorShaftRho=motor.shaftDensity  pulleyRho=pulley.density  spoolRho=spool.density  ringRho=ring.density  frameColor=frame.color  bracketColor=bracket.color  pinColor=frame.pinColor  motorHousingColor=motor.housingColor  motorFlangeColor=motor.flangeColor  motorShaftColor=motor.shaftColor  pulleyColor=pulley.color  pulleyMarkerColor=pulley.markerColor  spoolColor=spool.color  spoolMarkerColor=spool.markerColor  cableColor=cable.color  ringColor=ring.color
      settings: SourceProductBaseCode=MS
  LRUE : PMIOPort  Side=Left
  RRUE : PMIOPort  Port=2  Side=Right
  LRLE : PMIOPort  Port=3  Side=Left
  RRLE : PMIOPort  Port=4  Side=Right
  LFUE : PMIOPort  Port=5  Side=Left
  RFUE : PMIOPort  Port=6  Side=Right
  LFLE : PMIOPort  Port=7  Side=Left
  RFLE : PMIOPort  Port=8  Side=Right
  B : PMIOPort  Port=9  Side=Left
  connections:
  Base/RConn2 -- Right-Front Cable Assembly/LConn1
  Right-Rear Cable Assembly/LConn1 -- Base/RConn1
  Left-Front Cable Assembly/LConn1 -- Base/LConn2
  RRUE/RConn1 -- Right-Rear Cable Assembly/RConn1
  RRLE/RConn1 -- Right-Rear Cable Assembly/RConn2
  Base/LConn1 -- Left-Rear Cable Assembly/LConn1
  RFLE/RConn1 -- Right-Front Cable Assembly/RConn2
  LRUE/RConn1 -- Left-Rear Cable Assembly/RConn1
  Left-Front Cable Assembly/RConn1 -- LFUE/RConn1
  RFUE/RConn1 -- Right-Front Cable Assembly/RConn1
  LRLE/RConn1 -- Left-Rear Cable Assembly/RConn2
  LFLE/RConn1 -- Left-Front Cable Assembly/RConn2
  B/RConn1 -- Base/LConn3

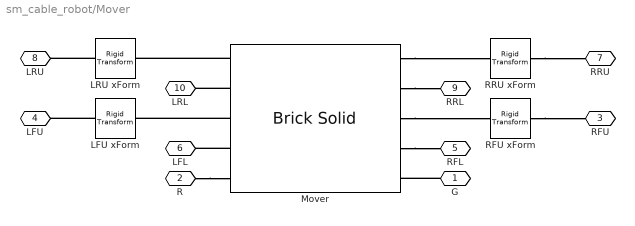
== system sm_cable_robot/Mover ==
  LFU xForm : sm_lib/Frames and Transforms/Rigid Transform  TranslationMethod=StandardAxis  TranslationStandardOffset=connectorOffset  TranslationLengthUnit=m  TranslationStandardAxis=+X  TranslationCartesianOffset=[0 0 0]  TranslationROffset=0  TranslationROffsetUnits=m  TranslationZOffset=0  TranslationZOffsetUnits=m  TranslationThetaOffset=0  TranslationThetaOffsetUnits=deg  RotationMethod=None  RotationAngleUnits=deg  RotationStandardAxis=+Z  RotationAngle=0.0  RotationArbitraryAxis=[0 0 1]  FollAlignAxisA=+X  BaseAlignAxisA=+Y  FollAlignAxisB=+Y  BaseAlignAxisB=+Z  RotationSequenceAxes=FollowerAxes  RotationSequence=XYX  RotationSequenceAngles=[0 0 0]  RotationSequenceAnglesUnits=deg  RotationMatrix=[1 0 0; 0 1 0; 0 0 1]
  LRU xForm : sm_lib/Frames and Transforms/Rigid Transform  TranslationMethod=StandardAxis  TranslationStandardOffset=connectorOffset  TranslationLengthUnit=m  TranslationStandardAxis=+X  TranslationCartesianOffset=[0 0 0]  TranslationROffset=0  TranslationROffsetUnits=m  TranslationZOffset=0  TranslationZOffsetUnits=m  TranslationThetaOffset=0  TranslationThetaOffsetUnits=deg  RotationMethod=None  RotationAngleUnits=deg  RotationStandardAxis=+Z  RotationAngle=0.0  RotationArbitraryAxis=[0 0 1]  FollAlignAxisA=+X  BaseAlignAxisA=+Y  FollAlignAxisB=+Y  BaseAlignAxisB=+Z  RotationSequenceAxes=FollowerAxes  RotationSequence=XYX  RotationSequenceAngles=[0 0 0]  RotationSequenceAnglesUnits=deg  RotationMatrix=[1 0 0; 0 1 0; 0 0 1]
  Mover : sm_lib/Body Elements/Brick Solid  GraphicAmbientColor=[0.15 0.15 0.15 1.0]  BasedOnType=Density  BrickDimensions=dimension  BrickDimensionUnits=m  CenterOfMass=[0 0 0]  CenterOfMassUnits=m  GraphicDiffuseColor=color  Density=rho  DensityUnits=kg/m^3  DoExposeReferenceFrame=off  GraphicEmissiveColor=[0.0 0.0 0.0 1.0]  ExportEntireGeometry=on  SerializedFrames=<Frames><Frame><Id>Frame1</Id><Value><Name>LRU</Name><Origin><Source>GeometricFeature</Source><FeatureName>-x +y +z point</FeatureName></Origin><PrimaryAxis><DefinedDirection>+Z</DefinedDirection><Source>ReferenceFrame</Source><SourceDirection>+Z</SourceDirection><FeatureName></FeatureName></PrimaryAxis><SecondaryAxis><DefinedDirection>+X</DefinedDirection><Source>ReferenceFrame</Source><SourceDirection>+X</SourceDirection><FeatureName></FeatureName></SecondaryAxis></Value></Frame><Frame><Id>Frame2</Id><Value><Name>RRU</Name><Origin><Source>GeometricFeature</Source><FeatureName>+x +y +z point</FeatureName></Origin><PrimaryAxis><DefinedDirection>+Z</DefinedDirection><Source>ReferenceFrame</Source><SourceDirection>+Z</SourceDirection><FeatureName></FeatureName></PrimaryAxis><SecondaryAxis><DefinedDirection>+X</DefinedDirection><Source>ReferenceFrame</Source><SourceDirection>+X</SourceDirection><FeatureName></FeatureName></SecondaryAxis></Value></Frame><Frame><Id>Frame3</Id><Value><Name>LRL</Name><Origin><Source>GeometricFeature</Source><FeatureName>-x +y -z point</FeatureName></Origin><PrimaryAxis><DefinedDirection>+Z</DefinedDirection><Source>ReferenceFrame</Source><SourceDirection>+Z</SourceDirection><FeatureName></FeatureName></PrimaryAxis><SecondaryAxis><DefinedDirection>+X</DefinedDirection><Source>ReferenceFrame</Source><SourceDirection>+X</SourceDirection><FeatureName></FeatureName></SecondaryAxis></Value></Frame><Frame><Id>Frame4</Id><Value><Name>RRL</Name><Origin><Source>GeometricFeature</Source><FeatureName>+x +y -z point</FeatureName></Origin><PrimaryAxis><DefinedDirection>+Z</DefinedDirection><Source>ReferenceFrame</Source><SourceDirection>+Z</SourceDirection><FeatureName></FeatureName></PrimaryAxis><SecondaryAxis><DefinedDirection>+X</DefinedDirection><Source>ReferenceFrame</Source><SourceDirection>+X</SourceDirection><FeatureName></FeatureName></SecondaryAxis></Value></Frame><Frame><Id>Frame5</Id><Value><Name>LFU</Name><Origin><Source>GeometricFeature</Source><FeatureName>-x -y +z point</FeatureName></Origin><PrimaryAxis><DefinedDirection>+Z</DefinedDirection><Source>ReferenceFrame</Source><SourceDirection>+Z</SourceDirection><FeatureName></FeatureName></PrimaryAxis><SecondaryAxis><DefinedDirection>+X</DefinedDirection><Source>ReferenceFrame</Source><SourceDirection>+X</SourceDirection><FeatureName></FeatureName></SecondaryAxis></Value></Frame><Frame><Id>Frame6</Id><Value><Name>RFU</Name><Origin><Source>GeometricFeature</Source><FeatureName>+x -y +z point</FeatureName></Origin><PrimaryAxis><DefinedDirection>+Z</DefinedDirection><Source>ReferenceFrame</Source><SourceDirection>+Z</SourceDirection><FeatureName></FeatureName></PrimaryAxis><SecondaryAxis><DefinedDirection>+X</DefinedDirection><Source>ReferenceFrame</Source><SourceDirection>+X</SourceDirection><FeatureName></FeatureName></SecondaryAxis></Value></Frame><Frame><Id>Frame7</Id><Value><Name>LFL</Name><Origin><Source>GeometricFeature</Source><FeatureName>-x -y -z point</FeatureName></Origin><PrimaryAxis><DefinedDirection>+Z</DefinedDirection><Source>ReferenceFrame</Source><SourceDirection>+Z</SourceDirection><FeatureName></FeatureName></PrimaryAxis><SecondaryAxis><DefinedDirection>+X</DefinedDirection><Source>ReferenceFrame</Source><SourceDirection>+X</SourceDirection><FeatureName></FeatureName></SecondaryAxis></Value></Frame><Frame><Id>Frame8</Id><Value><Name>RFL</Name><Origin><Source>GeometricFeature</Source><FeatureName>+x -y -z point</FeatureName></Origin><PrimaryAxis><DefinedDirection>+Z</DefinedDirection><Source>ReferenceFrame</Source><SourceDirection>+Z</SourceDirection><FeatureName></FeatureName></PrimaryAxis><SecondaryAxis><DefinedDirection>+X</DefinedDirection><Source>ReferenceFrame</Source><SourceDirection>+X</SourceDirection><FeatureName></FeatureName></SecondaryAxis></Value></Frame><Frame><Id>Frame9</Id><Value><Name>R</Name><Origin><Source>ReferenceFrame</Source><FeatureName></FeatureName></Origin><PrimaryAxis><DefinedDirection>+Z</DefinedDirection><Source>ReferenceFrame</Source><SourceDirection>+Z</SourceDirection><FeatureName></FeatureName></PrimaryAxis><SecondaryAxis><DefinedDirection>+X</DefinedDirection><Source>ReferenceFrame</Source><SourceDirection>+X</SourceDirection><FeatureName></FeatureName></SecondaryAxis></Value></Frame></Frames>  MarkerShape=Sphere  MarkerSize=10  GraphicType=FromGeometry  InertiaType=CalculateFromGeometry  Mass=1  MassUnits=kg  MomentsOfInertia=[1 1 1]  MomentsOfInertiaUnits=kg*m^2  GraphicOpacity=1.0  ProductsOfInertia=[0 0 0]  ProductsOfInertiaUnits=kg*m^2  GraphicShininess=75  GraphicSpecularColor=[0.5 0.5 0.5 1.0]  GraphicVisPropType=SimpleVisualProperties
  RFU xForm : sm_lib/Frames and Transforms/Rigid Transform  TranslationMethod=StandardAxis  TranslationStandardOffset=connectorOffset  TranslationLengthUnit=m  TranslationStandardAxis=-X  TranslationCartesianOffset=[0 0 0]  TranslationROffset=0  TranslationROffsetUnits=m  TranslationZOffset=0  TranslationZOffsetUnits=m  TranslationThetaOffset=0  TranslationThetaOffsetUnits=deg  RotationMethod=None  RotationAngleUnits=deg  RotationStandardAxis=+Z  RotationAngle=0.0  RotationArbitraryAxis=[0 0 1]  FollAlignAxisA=+X  BaseAlignAxisA=+Y  FollAlignAxisB=+Y  BaseAlignAxisB=+Z  RotationSequenceAxes=FollowerAxes  RotationSequence=XYX  RotationSequenceAngles=[0 0 0]  RotationSequenceAnglesUnits=deg  RotationMatrix=[1 0 0; 0 1 0; 0 0 1]
  RRU xForm : sm_lib/Frames and Transforms/Rigid Transform  TranslationMethod=StandardAxis  TranslationStandardOffset=connectorOffset  TranslationLengthUnit=m  TranslationStandardAxis=-X  TranslationCartesianOffset=[0 0 0]  TranslationROffset=0  TranslationROffsetUnits=m  TranslationZOffset=0  TranslationZOffsetUnits=m  TranslationThetaOffset=0  TranslationThetaOffsetUnits=deg  RotationMethod=None  RotationAngleUnits=deg  RotationStandardAxis=+Z  RotationAngle=0.0  RotationArbitraryAxis=[0 0 1]  FollAlignAxisA=+X  BaseAlignAxisA=+Y  FollAlignAxisB=+Y  BaseAlignAxisB=+Z  RotationSequenceAxes=FollowerAxes  RotationSequence=XYX  RotationSequenceAngles=[0 0 0]  RotationSequenceAnglesUnits=deg  RotationMatrix=[1 0 0; 0 1 0; 0 0 1]
  G : PMIOPort  Side=Right
  R : PMIOPort  Port=2  Side=Right
  RFU : PMIOPort  Port=3  Side=Right
  LFU : PMIOPort  Port=4  Side=Left
  RFL : PMIOPort  Port=5  Side=Right
  LFL : PMIOPort  Port=6  Side=Left
  RRU : PMIOPort  Port=7  Side=Right
  LRU : PMIOPort  Port=8  Side=Left
  RRL : PMIOPort  Port=9  Side=Right
  LRL : PMIOPort  Port=10  Side=Left
  connections:
  R/RConn1 -- Mover/LConn5
  LRU xForm/RConn1 -- LRU/RConn1
  Mover/LConn2 -- LRL/RConn1
  LFU xForm/RConn1 -- LFU/RConn1
  Mover/LConn4 -- LFL/RConn1
  RRU xForm/RConn1 -- RRU/RConn1
  Mover/RConn2 -- RRL/RConn1
  RFU xForm/RConn1 -- RFU/RConn1
  Mover/RConn4 -- RFL/RConn1
  Mover/LConn1 -- LRU xForm/LConn1
  Mover/LConn3 -- LFU xForm/LConn1
  Mover/RConn1 -- RRU xForm/LConn1
  Mover/RConn3 -- RFU xForm/LConn1
  G/RConn1 -- Mover/RConn5

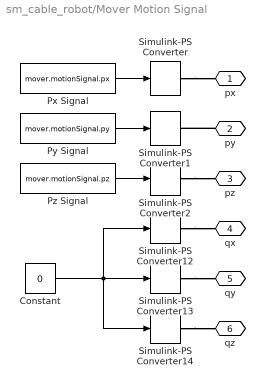
== system sm_cable_robot/Mover Motion Signal ==
  Constant : Constant  Value=0
  Px Signal : FromWorkspace  VariableName=mover.motionSignal.px  ZeroCross=off  OutputAfterFinalValue=Holding final value
  Py Signal : FromWorkspace  VariableName=mover.motionSignal.py  ZeroCross=off  OutputAfterFinalValue=Holding final value
  Pz Signal : FromWorkspace  VariableName=mover.motionSignal.pz  ZeroCross=off  OutputAfterFinalValue=Holding final value
  Simulink-PS Converter : nesl_utility/Simulink-PS Converter  PhysicalDomain=network_engine_domain  SubClassName=ps_input  LeftPortType=input  RightPortType=output  PseudoPeriodic=off  Frequencies=[]  NoiseDistribution=none  NoiseParameters=[]  Unit=1  AffineConversion=off  FilteringAndDerivatives=filter  SimscapeFilterOrder=2  InputFilterTimeConstant=mover.motionSignal.t_c  UdotUserProvided=2
      settings: SourceProductBaseCode=PW,SS
  Simulink-PS Converter1 : nesl_utility/Simulink-PS Converter  PhysicalDomain=network_engine_domain  SubClassName=ps_input  LeftPortType=input  RightPortType=output  PseudoPeriodic=off  Frequencies=[]  NoiseDistribution=none  NoiseParameters=[]  Unit=1  AffineConversion=off  FilteringAndDerivatives=filter  SimscapeFilterOrder=2  InputFilterTimeConstant=mover.motionSignal.t_c  UdotUserProvided=2
      settings: SourceProductBaseCode=PW,SS
  Simulink-PS Converter12 : nesl_utility/Simulink-PS Converter  PhysicalDomain=network_engine_domain  SubClassName=ps_input  LeftPortType=input  RightPortType=output  PseudoPeriodic=off  Frequencies=[]  NoiseDistribution=none  NoiseParameters=[]  Unit=1  AffineConversion=off  FilteringAndDerivatives=zero  SimscapeFilterOrder=2  InputFilterTimeConstant=mover.motionSignal.t_c  UdotUserProvided=0
      settings: SourceProductBaseCode=PW,SS
  Simulink-PS Converter13 : nesl_utility/Simulink-PS Converter  PhysicalDomain=network_engine_domain  SubClassName=ps_input  LeftPortType=input  RightPortType=output  PseudoPeriodic=off  Frequencies=[]  NoiseDistribution=none  NoiseParameters=[]  Unit=1  AffineConversion=off  FilteringAndDerivatives=zero  SimscapeFilterOrder=2  InputFilterTimeConstant=mover.motionSignal.t_c  UdotUserProvided=0
      settings: SourceProductBaseCode=PW,SS
  Simulink-PS Converter14 : nesl_utility/Simulink-PS Converter  PhysicalDomain=network_engine_domain  SubClassName=ps_input  LeftPortType=input  RightPortType=output  PseudoPeriodic=off  Frequencies=[]  NoiseDistribution=none  NoiseParameters=[]  Unit=1  AffineConversion=off  FilteringAndDerivatives=zero  SimscapeFilterOrder=2  InputFilterTimeConstant=mover.motionSignal.t_c  UdotUserProvided=0
      settings: SourceProductBaseCode=PW,SS
  Simulink-PS Converter2 : nesl_utility/Simulink-PS Converter  PhysicalDomain=network_engine_domain  SubClassName=ps_input  LeftPortType=input  RightPortType=output  PseudoPeriodic=off  Frequencies=[]  NoiseDistribution=none  NoiseParameters=[]  Unit=1  AffineConversion=off  FilteringAndDerivatives=filter  SimscapeFilterOrder=2  InputFilterTimeConstant=mover.motionSignal.t_c  UdotUserProvided=2
      settings: SourceProductBaseCode=PW,SS
  px : PMIOPort  Side=Right
  py : PMIOPort  Port=2  Side=Right
  pz : PMIOPort  Port=3  Side=Right
  qx : PMIOPort  Port=4  Side=Right
  qy : PMIOPort  Port=5  Side=Right
  qz : PMIOPort  Port=6  Side=Right
  wires:
  Px Signal/1 -> Simulink-PS Converter/1
  Py Signal/1 -> Simulink-PS Converter1/1
  Pz Signal/1 -> Simulink-PS Converter2/1
  Constant/1 -> Simulink-PS Converter14/1, Simulink-PS Converter13/1, Simulink-PS Converter12/1
  connections:
  Simulink-PS Converter2/RConn1 -- pz/RConn1
  py/RConn1 -- Simulink-PS Converter1/RConn1
  Simulink-PS Converter/RConn1 -- px/RConn1
  Simulink-PS Converter14/RConn1 -- qz/RConn1
  Simulink-PS Converter13/RConn1 -- qy/RConn1
  Simulink-PS Converter12/RConn1 -- qx/RConn1
